simulink model "SWC_TRSP"  (R2020a)
settings: Solver=FixedStepDiscrete  StartTime=0.0  StopTime=0.15  FixedStep=0.0001  RelTol=1e-3
values from neighbouring files (symbols this model uses):
  CAL_TRSP_18VHSVoltCountTrh_s16 = 0.0    [SWC_TRSP_DataDictionary.sldd]
  CAL_TRSP_18VHSVoltDebTrh_s16 = 0.0    [SWC_TRSP_DataDictionary.sldd]
  CAL_TRSP_18VHSVoltErrRst_b = 0.0    [SWC_TRSP_DataDictionary.sldd]
  CAL_TRSP_18VHSVoltHiLim_u16 = 0.0    [SWC_TRSP_DataDictionary.sldd]
  CAL_TRSP_18VHSVoltLoLim_u16 = 0.0    [SWC_TRSP_DataDictionary.sldd]
  CAL_TRSP_1V8CPLDVoltCountTrh_s16 = 0.0    [SWC_TRSP_DataDictionary.sldd]
  CAL_TRSP_1V8CPLDVoltDebTrh_s16 = 0.0    [SWC_TRSP_DataDictionary.sldd]
  CAL_TRSP_1V8CPLDVoltErrRst_b = 0.0    [SWC_TRSP_DataDictionary.sldd]
  CAL_TRSP_1V8CPLDVoltHiLim_u16 = 0.0    [SWC_TRSP_DataDictionary.sldd]
  CAL_TRSP_1V8CPLDVoltLoLim_u16 = 0.0    [SWC_TRSP_DataDictionary.sldd]
  CAL_TRSP_3V3CPLDVoltCountTrh_s16 = 0.0    [SWC_TRSP_DataDictionary.sldd]
  CAL_TRSP_3V3CPLDVoltDebTrh_s16 = 0.0    [SWC_TRSP_DataDictionary.sldd]
  CAL_TRSP_3V3CPLDVoltErrRst_b = 0.0    [SWC_TRSP_DataDictionary.sldd]
  CAL_TRSP_3V3CPLDVoltHiLim_u16 = 0.0    [SWC_TRSP_DataDictionary.sldd]
  CAL_TRSP_3V3CPLDVoltLoLim_u16 = 0.0    [SWC_TRSP_DataDictionary.sldd]
  CAL_TRSP_AgTimecompCtl_u8 = 0.0    [SWC_TRSP_DataDictionary.sldd]
  CAL_TRSP_CurrRngCountTrh_s16 = 0.0    [SWC_TRSP_DataDictionary.sldd]
  CAL_TRSP_CurrRngDebTrh_s16 = 0.0    [SWC_TRSP_DataDictionary.sldd]
  CAL_TRSP_CurrRngErrRst_b = 0.0    [SWC_TRSP_DataDictionary.sldd]
  CAL_TRSP_CurrSumCountTrh_s16 = 0.0    [SWC_TRSP_DataDictionary.sldd]
  CAL_TRSP_CurrSumDebTrh_s16 = 0.0    [SWC_TRSP_DataDictionary.sldd]
  CAL_TRSP_CurrSumErrRst_b = 0.0    [SWC_TRSP_DataDictionary.sldd]
  CAL_TRSP_CurrSumLim_f32 = 0.0    [SWC_TRSP_DataDictionary.sldd]
  CAL_TRSP_Diff_UBR_SBCLim_f32 = 0.0    [SWC_TRSP_DataDictionary.sldd]
  CAL_TRSP_flgChangPha_b = 0.0    [SWC_TRSP_DataDictionary.sldd]
  CAL_TRSP_iPhasSensVoltCountTrh_s16 = 0.0    [SWC_TRSP_DataDictionary.sldd]
  CAL_TRSP_iPhasSensVoltDebTrh_s16 = 0.0    [SWC_TRSP_DataDictionary.sldd]
  CAL_TRSP_iPhasSensVoltErrRst_b = 0.0    [SWC_TRSP_DataDictionary.sldd]
  CAL_TRSP_iPhasSensVoltHiLim_u16 = 0.0    [SWC_TRSP_DataDictionary.sldd]
  CAL_TRSP_iPhasSensVoltLoLim_u16 = 0.0    [SWC_TRSP_DataDictionary.sldd]
  CAL_TRSP_iPhaUOffset_f32 = 0.0    [SWC_TRSP_DataDictionary.sldd]
  CAL_TRSP_iPhaVOffset_f32 = 0.0    [SWC_TRSP_DataDictionary.sldd]
  CAL_TRSP_iPhaWOffset_f32 = 0.0    [SWC_TRSP_DataDictionary.sldd]
  CAL_TRSP_iUCnvFac_f32 = 0.0    [SWC_TRSP_DataDictionary.sldd]
  CAL_TRSP_iVCnvFac_f32 = 0.0    [SWC_TRSP_DataDictionary.sldd]
  CAL_TRSP_iWCnvFac_f32 = 0.0    [SWC_TRSP_DataDictionary.sldd]
  CAL_TRSP_OfstErrRst_b = 0.0    [SWC_TRSP_DataDictionary.sldd]
  CAL_TRSP_OfstRngHiLim_f32 = 0.0    [SWC_TRSP_DataDictionary.sldd]
  CAL_TRSP_OfstRngLoLim_f32 = 0.0    [SWC_TRSP_DataDictionary.sldd]
  CAL_TRSP_ReqTrqCountTrh_s16 = 0.0    [SWC_TRSP_DataDictionary.sldd]
  CAL_TRSP_ReqTrqDebTrh_s16 = 0.0    [SWC_TRSP_DataDictionary.sldd]
  CAL_TRSP_ReqTrqErrRst_b = 0.0    [SWC_TRSP_DataDictionary.sldd]
  CAL_TRSP_ReqTrqHiLim_f32 = 0.0    [SWC_TRSP_DataDictionary.sldd]
  CAL_TRSP_ReqTrqLoLim_f32 = 0.0    [SWC_TRSP_DataDictionary.sldd]
  CAL_TRSP_RslvExciCountTrh_s16 = 0.0    [SWC_TRSP_DataDictionary.sldd]
  CAL_TRSP_RslvExciDebTrh_s16 = 0.0    [SWC_TRSP_DataDictionary.sldd]
  CAL_TRSP_RslvExciErrRst_b = 0.0    [SWC_TRSP_DataDictionary.sldd]
  CAL_TRSP_RslvMaxSele_u8 = 0.0    [SWC_TRSP_DataDictionary.sldd]
  CAL_TRSP_RslvMinSele_u8 = 0.0    [SWC_TRSP_DataDictionary.sldd]
  CAL_TRSP_RslvRngCosNHiLim_u16 = 0.0    [SWC_TRSP_DataDictionary.sldd]
  CAL_TRSP_RslvRngCosNLoLim_u16 = 0.0    [SWC_TRSP_DataDictionary.sldd]
  CAL_TRSP_RslvRngCosPHiLim_u16 = 0.0    [SWC_TRSP_DataDictionary.sldd]
  CAL_TRSP_RslvRngCosPLoLim_u16 = 0.0    [SWC_TRSP_DataDictionary.sldd]
  CAL_TRSP_RslvRngCountTrh_s16 = 0.0    [SWC_TRSP_DataDictionary.sldd]
  CAL_TRSP_RslvRngDebTrh_s16 = 0.0    [SWC_TRSP_DataDictionary.sldd]
  CAL_TRSP_RslvRngErrRst_b = 0.0    [SWC_TRSP_DataDictionary.sldd]
  CAL_TRSP_RslvRngExciHiLim_u16 = 0.0    [SWC_TRSP_DataDictionary.sldd]
  CAL_TRSP_RslvRngExciLoLim_u16 = 0.0    [SWC_TRSP_DataDictionary.sldd]
  CAL_TRSP_RslvRngSinNHiLim_u16 = 0.0    [SWC_TRSP_DataDictionary.sldd]
  CAL_TRSP_RslvRngSinNLoLim_u16 = 0.0    [SWC_TRSP_DataDictionary.sldd]
  CAL_TRSP_RslvRngSinPHiLim_u16 = 0.0    [SWC_TRSP_DataDictionary.sldd]
  CAL_TRSP_RslvRngSinPLoLim_u16 = 0.0    [SWC_TRSP_DataDictionary.sldd]
  CAL_TRSP_RslvSensVoltCountTrh_s16 = 0.0    [SWC_TRSP_DataDictionary.sldd]
  CAL_TRSP_RslvSensVoltDebTrh_s16 = 0.0    [SWC_TRSP_DataDictionary.sldd]
  CAL_TRSP_RslvSensVoltErrRst_b = 0.0    [SWC_TRSP_DataDictionary.sldd]
  CAL_TRSP_RslvSensVoltHiLim_u16 = 0.0    [SWC_TRSP_DataDictionary.sldd]
  CAL_TRSP_RslvSensVoltLoLim_u16 = 0.0    [SWC_TRSP_DataDictionary.sldd]
  CAL_TRSP_RslvSqrtCountTrh_s16 = 0.0    [SWC_TRSP_DataDictionary.sldd]
  CAL_TRSP_RslvSqrtDebTrh_s16 = 0.0    [SWC_TRSP_DataDictionary.sldd]
  CAL_TRSP_RslvSqrtErrRst_b = 0.0    [SWC_TRSP_DataDictionary.sldd]
  CAL_TRSP_RslvSqrtHiLim_u16 = 0.0    [SWC_TRSP_DataDictionary.sldd]
  CAL_TRSP_RslvSqrtLoLim_u16 = 0.0    [SWC_TRSP_DataDictionary.sldd]
  CAL_TRSP_SpeedCtlMode_u8 = 0.0    [SWC_TRSP_DataDictionary.sldd]
  CAL_TRSP_TorqueCtlMode_u8 = 0.0    [SWC_TRSP_DataDictionary.sldd]
  CAL_TRSP_UB_SBCCnvFac_f32 = 0.0    [SWC_TRSP_DataDictionary.sldd]
  CAL_TRSP_UBRVoltCountTrh_s16 = 0.0    [SWC_TRSP_DataDictionary.sldd]
  CAL_TRSP_UBRVoltDebTrh_s16 = 0.0    [SWC_TRSP_DataDictionary.sldd]
  CAL_TRSP_UBRVoltErrRst_b = 0.0    [SWC_TRSP_DataDictionary.sldd]
  CAL_TRSP_UBRWIDECnvFac_f32 = 0.0    [SWC_TRSP_DataDictionary.sldd]
  CAL_TRSP_UCurrRngHiLim_f32 = 0.0    [SWC_TRSP_DataDictionary.sldd]
  CAL_TRSP_UCurrRngLoLim_f32 = 0.0    [SWC_TRSP_DataDictionary.sldd]
  CAL_TRSP_VCurrRngHiLim_f32 = 0.0    [SWC_TRSP_DataDictionary.sldd]
  CAL_TRSP_VCurrRngLoLim_f32 = 0.0    [SWC_TRSP_DataDictionary.sldd]
  CAL_TRSP_WCurrRngHiLim_f32 = 0.0    [SWC_TRSP_DataDictionary.sldd]
  CAL_TRSP_WCurrRngLoLim_f32 = 0.0    [SWC_TRSP_DataDictionary.sldd]
  GLB_TRSP_CircAge_f32 = 0.0    [SWC_TRSP_DataDictionary.sldd]
  GLB_TRSP_MotorPole_u8 = 0.0    [SWC_TRSP_DataDictionary.sldd]
  GLB_TRSP_Sixty_f32 = 0.0    [SWC_TRSP_DataDictionary.sldd]
libraries: simulink x22
(part 2 of 13)

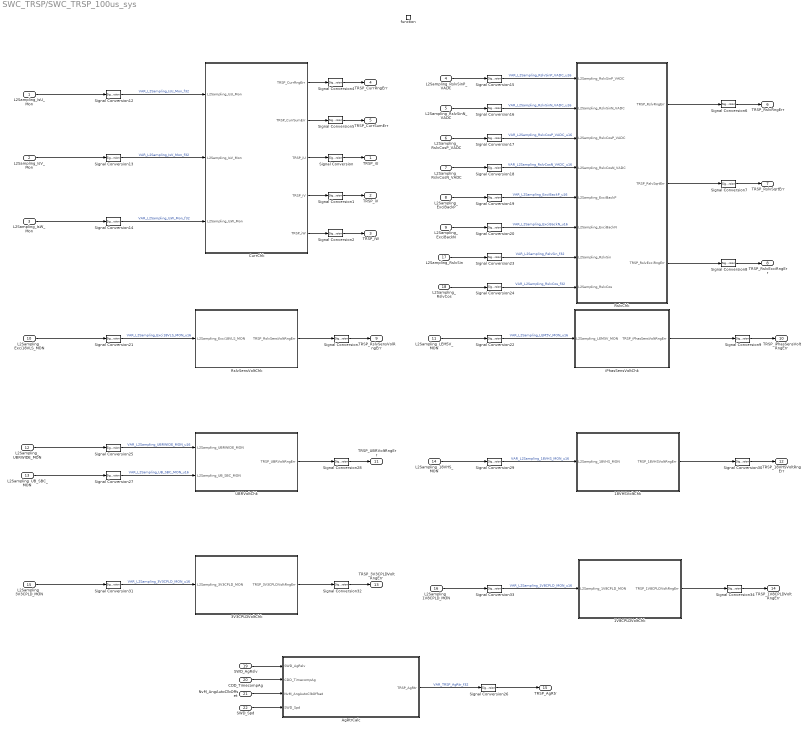
== system SWC_TRSP/SWC_TRSP_100us_sys ==
  L2Sampling_IsU_Mon : Inport
  L2Sampling_IsV_Mon : Inport  Port=2
  L2Sampling_IsW_Mon : Inport  Port=3
  L2Sampling_RslvSinP_VADC : Inport  Port=4
  L2Sampling_RslvSinN_VADC : Inport  Port=5
  L2Sampling_RslvCosP_VADC : Inport  Port=6
  L2Sampling_RslvCosN_VADC : Inport  Port=7
  L2Sampling_ExciBackP : Inport  Port=8
  L2Sampling_ExciBackN : Inport  Port=9
  L2Sampling_Exci18VLS_MON : Inport  Port=10
  L2Sampling_LEM5V_MON : Inport  Port=11
  L2Sampling_UBRWIDE_MON : Inport  Port=12
  L2Sampling_UB_SBC_MON : Inport  Port=13
  L2Sampling_18VHS_MON : Inport  Port=14
  L2Sampling_3V3CPLD_MON : Inport  Port=15
  L2Sampling_1V8CPLD_MON : Inport  Port=16
  L2Sampling_RslvSin : Inport  Port=17
  L2Sampling_RslvCos : Inport  Port=18
  SWD_AgRslv : Inport  Port=19
  CDD_TimecompAg : Inport  Port=20
  NvM_AngAutoClbOffset : Inport  Port=21
  SWD_Spd : Inport  Port=22
  function : TriggerPort  TriggerType=function-call  VariantControl=(inherit)  SampleTimeType=periodic  SampleTime=-1
  18VHSVoltChk : Subsystem
  1V8CPLDVoltChk : Subsystem
  3V3CPLDVoltChk : Subsystem
  AgRtrCalc : Subsystem  TreatAsAtomicUnit=on
      settings: RTWSystemCode=Nonreusable function
  CurrChk : Subsystem
      settings: RTWSystemCode=Nonreusable function
  RslvChk : Subsystem
  RslvSensVoltChk : Subsystem
  Signal Conversion{,1..9,12..34} (33 alike) : SignalConversion  OverrideOpt=off
  UBRVoltChk : Subsystem
  iPhasSensVoltChk : Subsystem
  TRSP_iU : Outport
  TRSP_iV : Outport  Port=2
  TRSP_iW : Outport  Port=3
  TRSP_CurrRngErr : Outport  Port=4
  TRSP_CurrSumErr : Outport  Port=5
  TRSP_RslvRngErr : Outport  Port=6
  TRSP_RslvSqrtErr : Outport  Port=7
  TRSP_RslvExciRngErr : Outport  Port=8
  TRSP_RslvSensVolRngErr : Outport  Port=9
  TRSP_iPhasSensVoltRngErr : Outport  Port=10
  TRSP_UBRVoltRngErr : Outport  Port=11
  TRSP_18VHSVoltRngErr : Outport  Port=12
  TRSP_3V3CPLDVoltRngErr : Outport  Port=13
  TRSP_1V8CPLDVoltRngErr : Outport  Port=14
  TRSP_AgRtr : Outport  Port=15  VectorParamsAs1DForOutWhenUnconnected=off
  wires:
  RslvChk/3(TRSP_RslvExciRngErr) -> Signal Conversion8/1
  RslvChk/2(TRSP_RslvSqrtErr) -> Signal Conversion7/1
  CurrChk/2(TRSP_CurrSumErr) -> Signal Conversion5/1
  RslvSensVoltChk/1(TRSP_RslvSensVoltRngErr) -> Signal Conversion3/1
  iPhasSensVoltChk/1(TRSP_iPhasSensVoltRngErr) -> Signal Conversion9/1
  L2Sampling_ExciBackN/1 -> Signal Conversion20/1
  L2Sampling_ExciBackP/1 -> Signal Conversion19/1
  CurrChk/1(TRSP_CurrRngErr) -> Signal Conversion4/1
  RslvChk/1(TRSP_RslvRngErr) -> Signal Conversion6/1
  L2Sampling_IsW_Mon/1 -> Signal Conversion14/1
  L2Sampling_IsU_Mon/1 -> Signal Conversion12/1
  L2Sampling_IsV_Mon/1 -> Signal Conversion13/1
  Signal Conversion/1 -> TRSP_iU/1
  Signal Conversion1/1 -> TRSP_iV/1
  Signal Conversion2/1 -> TRSP_iW/1
  Signal Conversion3/1 -> TRSP_RslvSensVolRngErr/1
  Signal Conversion4/1 -> TRSP_CurrRngErr/1
  Signal Conversion5/1 -> TRSP_CurrSumErr/1
  Signal Conversion6/1 -> TRSP_RslvRngErr/1
  Signal Conversion7/1 -> TRSP_RslvSqrtErr/1
  Signal Conversion8/1 -> TRSP_RslvExciRngErr/1
  Signal Conversion9/1 -> TRSP_iPhasSensVoltRngErr/1
  CurrChk/3(TRSP_iU) -> Signal Conversion/1
  CurrChk/5(TRSP_iW) -> Signal Conversion2/1
  CurrChk/4(TRSP_iV) -> Signal Conversion1/1
  L2Sampling_RslvSinP_VADC/1 -> Signal Conversion15/1
  L2Sampling_RslvSinN_VADC/1 -> Signal Conversion16/1
  L2Sampling_RslvCosP_VADC/1 -> Signal Conversion17/1
  L2Sampling_RslvCosN_VADC/1 -> Signal Conversion18/1
  Signal Conversion12/1 -> CurrChk/1(L2Sampling_IsU_Mon)  "VAR_L2Sampling_IsU_Mon_f32"
  Signal Conversion13/1 -> CurrChk/2(L2Sampling_IsV_Mon)  "VAR_L2Sampling_IsV_Mon_f32"
  Signal Conversion14/1 -> CurrChk/3(L2Sampling_IsW_Mon)  "VAR_L2Sampling_IsW_Mon_f32"
  Signal Conversion15/1 -> RslvChk/1(L2Sampling_RslvSinP_VADC)  "VAR_L2Sampling_RslvSinP_VADC_u16"
  Signal Conversion16/1 -> RslvChk/2(L2Sampling_RslvSinN_VADC)  "VAR_L2Sampling_RslvSinN_VADC_u16"
  Signal Conversion17/1 -> RslvChk/3(L2Sampling_RslvCosP_VADC)  "VAR_L2Sampling_RslvCosP_VADC_u16"
  Signal Conversion18/1 -> RslvChk/4(L2Sampling_RslvCosN_VADC)  "VAR_L2Sampling_RslvCosN_VADC_u16"
  Signal Conversion19/1 -> RslvChk/5(L2Sampling_ExciBackP)  "VAR_L2Sampling_ExciBackP_u16"
  Signal Conversion20/1 -> RslvChk/6(L2Sampling_ExciBackN)  "VAR_L2Sampling_ExciBackN_u16"
  Signal Conversion21/1 -> RslvSensVoltChk/1(L2Sampling_Exci18VLS_MON)  "VAR_L2Sampling_Exci18VLS_MON_u16"
  Signal Conversion22/1 -> iPhasSensVoltChk/1(L2Sampling_LEM5V_MON)  "VAR_L2Sampling_LEM5V_MON_u16"
  L2Sampling_Exci18VLS_MON/1 -> Signal Conversion21/1
  L2Sampling_LEM5V_MON/1 -> Signal Conversion22/1
  L2Sampling_UBRWIDE_MON/1 -> Signal Conversion25/1
  Signal Conversion27/1 -> UBRVoltChk/2(L2Sampling_UB_SBC_MON)  "VAR_L2Sampling_UB_SBC_MON_u16"
  Signal Conversion25/1 -> UBRVoltChk/1(L2Sampling_UBRWIDE_MON)  "VAR_L2Sampling_UBRWIDE_MON_u16"
  3V3CPLDVoltChk/1(TRSP_3V3CPLDVoltRngErr) -> Signal Conversion32/1
  L2Sampling_UB_SBC_MON/1 -> Signal Conversion27/1
  Signal Conversion30/1 -> TRSP_18VHSVoltRngErr/1
  Signal Conversion31/1 -> 3V3CPLDVoltChk/1(L2Sampling_3V3CPLD_MON)  "VAR_L2Sampling_3V3CPLD_MON_u16"
  18VHSVoltChk/1(TRSP_18VHSVoltRngErr) -> Signal Conversion30/1
  Signal Conversion32/1 -> TRSP_3V3CPLDVoltRngErr/1
  Signal Conversion29/1 -> 18VHSVoltChk/1(L2Sampling_18VHS_MON)  "VAR_L2Sampling_18VHS_MON_u16"
  UBRVoltChk/1(TRSP_UBRVoltRngErr) -> Signal Conversion28/1
  1V8CPLDVoltChk/1(TRSP_1V8CPLDVoltRngErr) -> Signal Conversion34/1
  L2Sampling_3V3CPLD_MON/1 -> Signal Conversion31/1
  Signal Conversion28/1 -> TRSP_UBRVoltRngErr/1
  L2Sampling_18VHS_MON/1 -> Signal Conversion29/1
  Signal Conversion34/1 -> TRSP_1V8CPLDVoltRngErr/1
  L2Sampling_1V8CPLD_MON/1 -> Signal Conversion33/1
  Signal Conversion33/1 -> 1V8CPLDVoltChk/1(L2Sampling_1V8CPLD_MON)  "VAR_L2Sampling_1V8CPLD_MON_u16"
  L2Sampling_RslvSin/1 -> Signal Conversion23/1
  L2Sampling_RslvCos/1 -> Signal Conversion24/1
  Signal Conversion23/1 -> RslvChk/7(L2Sampling_RslvSin)  "VAR_L2Sampling_RslvSin_f32"
  Signal Conversion24/1 -> RslvChk/8(L2Sampling_RslvCos)  "VAR_L2Sampling_RslvCos_f32"
  NvM_AngAutoClbOffset/1 -> AgRtrCalc/3(NvM_AngAutoClbOffset)
  SWD_AgRslv/1 -> AgRtrCalc/1(SWD_AgRslv)
  CDD_TimecompAg/1 -> AgRtrCalc/2(CDD_TimecompAg)
  SWD_Spd/1 -> AgRtrCalc/4(SWD_Spd)
  Signal Conversion26/1 -> TRSP_AgRtr/1
  AgRtrCalc/1(TRSP_AgRtr) -> Signal Conversion26/1  "VAR_TRSP_AgRtr_f32"

== system SWC_TRSP/SWC_TRSP_10ms_sys ==
  L2Com_TrqSetP : Inport  PortDimensions=1
  function : TriggerPort  TriggerType=function-call  VariantControl=(inherit)  SampleTimeType=periodic  SampleTime=-1
  CANSigChk : Subsystem
  Debouncer : Subsystem  Commented=on  TreatAsAtomicUnit=on
  Ground{,1..3} (4 alike) : Ground  Commented=on
  Signal Conversion3 : SignalConversion  OverrideOpt=off
  Signal Conversion7 : SignalConversion  OverrideOpt=off
  Terminator : Terminator  Commented=on
  Terminator1 : Terminator  Commented=on
  Terminator2 : Terminator  Commented=on
  TRSP_TrqSetPRngErr : Outport
  wires:
  Signal Conversion7/1 -> CANSigChk/1(L2Com_TrqSetP)  "VAR_L2Com_TrqSetP_f32"
  Debouncer/1(OutLock) -> Terminator/1
  Ground2/1 -> Debouncer/3(CountTrh)
  Ground/1 -> Debouncer/1(BooleanIN)
  Debouncer/3(Deb) -> Terminator2/1
  Ground1/1 -> Debouncer/2(Rst)
  Debouncer/2(Count) -> Terminator1/1
  Ground3/1 -> Debouncer/4(DebTrh)
  CANSigChk/1(TRSP_TrqSetPRngErr) -> Signal Conversion3/1
  L2Com_TrqSetP/1 -> Signal Conversion7/1
  Signal Conversion3/1 -> TRSP_TrqSetPRngErr/1

== system SWC_TRSP/SWC_TRSP_1ms_sys ==
  L2Com_ModeReq : Inport  PortDimensions=1
  NvM_AngAutoClbOffset : Inport  Port=2
  function : TriggerPort  TriggerType=function-call  VariantControl=(inherit)  SampleTimeType=periodic  SampleTime=-1
  Debouncer : Subsystem  Commented=on  TreatAsAtomicUnit=on
  Ground{,1..3} (4 alike) : Ground  Commented=on
  OfstAgChk : Subsystem
  Signal Conversion : SignalConversion  OverrideOpt=off
  Signal Conversion1 : SignalConversion  OverrideOpt=off
  Signal Conversion4 : SignalConversion  OverrideOpt=off
  Terminator : Terminator  Commented=on
  Terminator1 : Terminator  Commented=on
  Terminator2 : Terminator  Commented=on
  TRSP_OfstRngErr : Outport
  wires:
  Signal Conversion/1 -> TRSP_OfstRngErr/1
  NvM_AngAutoClbOffset/1 -> Signal Conversion4/1
  OfstAgChk/1(TRSP_OfstRngErr) -> Signal Conversion/1
  Ground3/1 -> Debouncer/4(DebTrh)
  Debouncer/2(Count) -> Terminator1/1
  Ground1/1 -> Debouncer/2(Rst)
  Debouncer/3(Deb) -> Terminator2/1
  Ground/1 -> Debouncer/1(BooleanIN)
  Ground2/1 -> Debouncer/3(CountTrh)
  Debouncer/1(OutLock) -> Terminator/1
  Signal Conversion4/1 -> OfstAgChk/2(NvM_AngAutoClbOffset)  "VAR_NvM_AngAutoClbOffset_f32"
  L2Com_ModeReq/1 -> Signal Conversion1/1
  Signal Conversion1/1 -> OfstAgChk/1(L2Com_ModeReq)  "VAR_L2Com_ModeReq_u16"

== system SWC_TRSP/SWC_TRSP_Init ==
  Event Listener : EventListener  EventName=reset

== system SWC_TRSP/SWC_TRSP_100us_sys/18VHSVoltChk ==
  L2Sampling_18VHS_MON : Inport
  CAL_TOM_CurrRngDebTrh_s1 : Constant  Value=CAL_TRSP_18VHSVoltDebTrh_s16  OutDataTypeStr=int16
  CAL_TOM_CurrRngDebTrh_s16 : Constant  Value=CAL_TRSP_18VHSVoltCountTrh_s16  OutDataTypeStr=int16
  CAL_TOM_CurrRngErrRst_b1 : Constant  Value=CAL_TRSP_18VHSVoltErrRst_b  OutDataTypeStr=boolean
  CAL_TOM_CurrRngHiLim_f32 : Constant  Value=CAL_TRSP_18VHSVoltHiLim_u16
  CAL_TOM_CurrRngLoLim_f32 : Constant  Value=CAL_TRSP_18VHSVoltLoLim_u16
  Debouncer11 : Subsystem  TreatAsAtomicUnit=on
  RngChk : Subsystem  TreatAsAtomicUnit=on
  TRSP_18VHSVoltRngErr : Outport
  wires:
  CAL_TOM_CurrRngErrRst_b1/1 -> Debouncer11/2(Rst)
  CAL_TOM_CurrRngDebTrh_s16/1 -> Debouncer11/3(CountTrh)
  CAL_TOM_CurrRngDebTrh_s1/1 -> Debouncer11/4(DebTrh)
  RngChk/1(TRSP_RngChkRslt) -> Debouncer11/1(BooleanIN)  "VAR_TRSP_18VHSVoltRngChkRslt_b"
  L2Sampling_18VHS_MON/1 -> RngChk/1(TRSP_RngChkVal)
  Debouncer11/1(OutLock) -> TRSP_18VHSVoltRngErr/1  "VAR_TRSP_18VHSVoltRngErr_b"
  CAL_TOM_CurrRngLoLim_f32/1 -> RngChk/3(TRSP_LoTrh)
  CAL_TOM_CurrRngHiLim_f32/1 -> RngChk/2(TRSP_HiTrh)
